simulink model "controlador"  (R2020b)
settings: Solver=VariableStepAuto  StartTime=0.0  StopTime=5  RelTol=1e-3
values from neighbouring files (symbols this model uses):
  K_area = 1.2    [K_tau_estimados.mat]
  tau_area = 0.1077    [K_tau_estimados.mat]    (also in exp4.m = tau_area(steptime,initialvalue,finalvalue,times,values))
undefined symbols (not defined in the file or in its folder): Kp, z
settings Model: Creator=lucas  LastModifiedBy=lucas

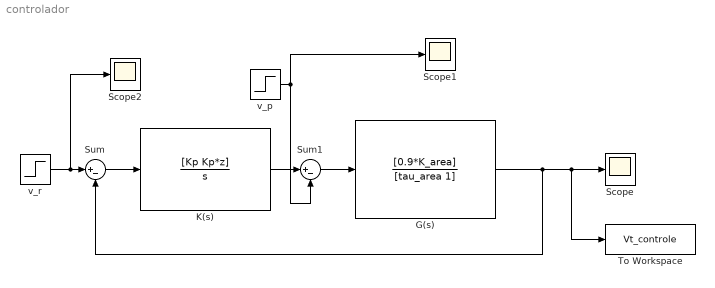
== system controlador ==
  G(s) : TransferFcn  Numerator=[0.9*K_area]  Denominator=[tau_area 1]
  K(s) : TransferFcn  Numerator=[Kp Kp*z]  Denominator=[1 0]
  Scope : Scope
  Scope1 : Scope
  Scope2 : Scope
  Sum : Sum  Inputs=|+-
  Sum1 : Sum  Inputs=|+-
  To Workspace : ToWorkspace  VariableName=Vt_controle  SaveFormat=Timeseries  SampleTime=-1
  v_p : Step  Time=3  SampleTime=0
  v_r : Step  Time=0  After=10  SampleTime=0
  wires:
  Sum/1 -> K(s)/1
  v_r/1 -> Scope2/1, Sum/1
  G(s)/1 -> To Workspace/1, Scope/1, Sum/2
  Sum1/1 -> G(s)/1
  K(s)/1 -> Sum1/1
  v_p/1 -> Scope1/1, Sum1/2
